simulink model "sampleModel2403_pp_difftest"  (R2018a)
settings: Solver=VariableStepAuto  StartTime=0.0  StopTime=10.0  RelTol=1e-3
undefined symbols (not defined in the file): DiscIntNeverNeededParam, sigbuilder_block
libraries: simulink x128
(part 3 of 3)

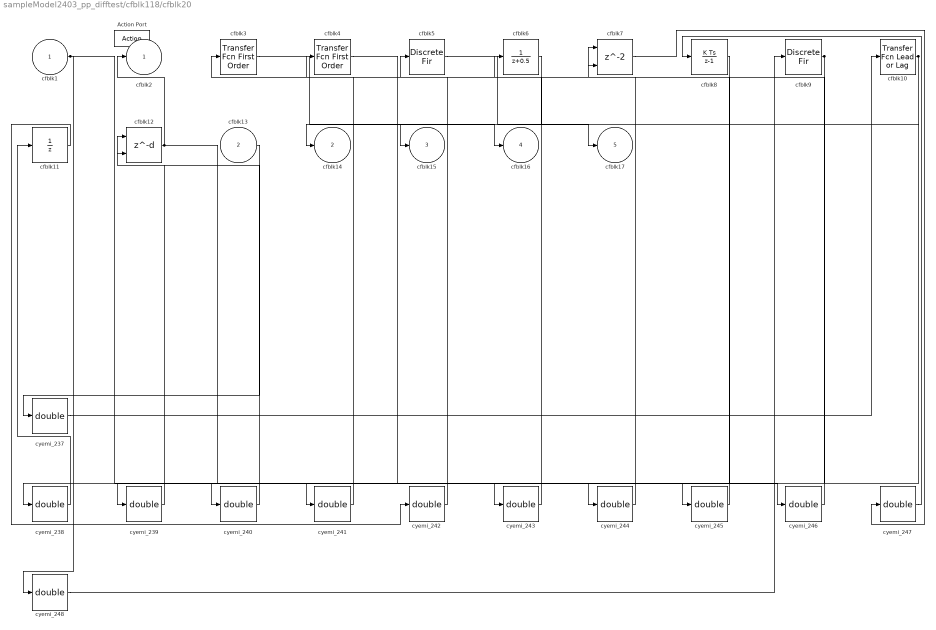
== system sampleModel2403_pp_difftest/cfblk118/cfblk20 ==
  cfblk1 : Inport
  cfblk13 : Inport  Port=2
  Action Port : ActionPort  ActionType=else
  cfblk10 : simulink/Discrete/Transfer Fcn Lead or Lag  PoleZ=0.95  ZeroZ=0.75  ICPrevOutput=0.0  ICPrevInput=0.0  DoSatur=off
      settings: SourceProductName=Simulink  SourceProductBaseCode=SL
  cfblk11 : UnitDelay  SampleTime=-1
  cfblk12 : Delay  DelayLengthSource=Input port
      settings: InputPortMap=u0,p1
  cfblk3 : simulink/Discrete/Transfer Fcn First Order  PoleZ=0.95  ICPrevOutput=0.0  DoSatur=off
      settings: SourceProductName=Simulink
  cfblk4 : simulink/Discrete/Transfer Fcn First Order  PoleZ=0.95  ICPrevOutput=0.0  DoSatur=off
      settings: SourceProductName=Simulink
  cfblk5 : DiscreteFir
  cfblk6 : DiscreteTransferFcn
  cfblk7 : Delay  ShowEnablePort=on
      settings: InputPortMap=u0,e6
  cfblk8 : DiscreteIntegrator  SampleTime=-1  OutDataTypeStr=double  ICPrevOutput=DiscIntNeverNeededParam  ICPrevScaledInput=DiscIntNeverNeededParam
  cfblk9 : DiscreteFir
  cyemi_{237..248} (12 alike) : DataTypeConversion  OutDataTypeStr=double
  cfblk2 : Outport
  cfblk14 : Outport  Port=2
  cfblk15 : Outport  Port=3
  cfblk16 : Outport  Port=4
  cfblk17 : Outport  Port=5
  wires:
  cfblk12/1 -> cfblk2/1, cyemi_243/1
  cfblk5/1 -> cfblk17/1
  cfblk3/1 -> cfblk16/1
  cfblk9/1 -> cyemi_239/1, cyemi_240/1, cyemi_241/1
  cfblk6/1 -> cfblk14/1
  cfblk10/1 -> cfblk15/1, cyemi_245/1
  cfblk1/1 -> cyemi_238/1, cyemi_246/1
  cyemi_237/1 -> cfblk10/1
  cfblk13/1 -> cyemi_237/1
  cyemi_238/1 -> cfblk11/1
  cyemi_239/1 -> cfblk12/1
  cyemi_240/1 -> cfblk12/2
  cyemi_241/1 -> cfblk3/1
  cyemi_242/1 -> cfblk4/1
  cfblk11/1 -> cyemi_242/1
  cyemi_243/1 -> cfblk5/1
  cyemi_244/1 -> cfblk6/1
  cfblk4/1 -> cyemi_244/1
  cyemi_245/1 -> cfblk7/1
  cyemi_246/1 -> cfblk7/2
  cyemi_247/1 -> cfblk8/1
  cfblk7/1 -> cyemi_247/1
  cyemi_248/1 -> cfblk9/1
  cfblk8/1 -> cyemi_248/1

== system sampleModel2403_pp_difftest/cfblk123/cfblk17 ==
  cfblk1 : Inport
  Action Port : ActionPort  ActionType=then
  cfblk10 : Delay
  cfblk3 : simulink/Discrete/Transfer Fcn Lead or Lag  PoleZ=0.95  ZeroZ=0.75  ICPrevOutput=0.0  ICPrevInput=0.0  DoSatur=off
      settings: SourceProductName=Simulink  SourceProductBaseCode=SL
  cfblk4 : UnitDelay  SampleTime=-1
  cfblk5 : simulink/Discrete/Transfer Fcn First Order  PoleZ=0.95  ICPrevOutput=0.0  DoSatur=off
      settings: SourceProductName=Simulink
  cfblk6 : simulink/Discrete/Transfer Fcn First Order  PoleZ=0.95  ICPrevOutput=0.0  DoSatur=off
      settings: SourceProductName=Simulink
  cfblk7 : DiscreteStateSpace  SampleTime=-1
  cfblk8 : simulink/Continuous/PID Controller  Controller=PID  TimeDomain=Discrete-time  SampleTime=-1  IntegratorMethod=Forward Euler  FilterMethod=Forward Euler  Form=Parallel  UseFilter=on  ControllerParametersSource=internal  P=1  I=1  D=0  N=100  InitialConditionSource=internal  InitialConditionForIntegrator=0  InitialConditionForFilter=0  ExternalReset=none  LimitOutput=off  UpperSaturationLimit=inf  LowerSaturationLimit=-inf  LinearizeAsGain=off  AntiWindupMode=none  Kb=1  TrackingMode=off  Kt=1  PParamMin=[]  PParamMax=[]  IParamMin=[]  IParamMax=[]  DParamMin=[]  DParamMax=[]  NParamMin=[]  NParamMax=[]  KbParamMin=[]  KbParamMax=[]  KtParamMin=[]  KtParamMax=[]  POutMin=[]  POutMax=[]  IOutMin=[]  IOutMax=[]  DOutMin=[]  DOutMax=[]  NOutMin=[]  NOutMax=[]  KbOutMin=[]  KbOutMax=[]  KtOutMin=[]  KtOutMax=[]  IntegratorOutMin=[]  IntegratorOutMax=[]  FilterOutMin=[]  FilterOutMax=[]  SumOutMin=[]  SumOutMax=[]  SumI1OutMin=[]  SumI1OutMax=[]  SumI2OutMin=[]  SumI2OutMax=[]  SumI3OutMin=[]  SumI3OutMax=[]  SumDOutMin=[]  SumDOutMax=[]  SaturationOutMin=[]  SaturationOutMax=[]  IntegratorContinuousStateAttributes=''  IntegratorStateMustResolveToSignalObject=off  IntegratorRTWStateStorageClass=Auto  FilterContinuousStateAttributes=''  FilterStateMustResolveToSignalObject=off  FilterRTWStateStorageClass=Auto  DifferentiatorICPrevScaledInput=0  DifferentiatorOutMin=[]  DifferentiatorOutMax=[]  FilterDiffOutCoefMin=[]  FilterDiffOutCoefMax=[]  SumDenOutMin=[]  SumDenOutMax=[]  SumNumOutMin=[]  SumNumOutMax=[]  ReciprocalOutMin=[]  ReciprocalOutMax=[]  DivideOutMin=[]  DivideOutMax=[]  TunerSelectOption=Transfer Function Based (PID Tuner App)
  cyemi_{334..340} (7 alike) : DataTypeConversion  OutDataTypeStr=double
  cfblk2 : Outport
  cfblk9 : Outport  Port=2
  wires:
  cfblk4/1 -> cfblk2/1
  cfblk6/1 -> cyemi_335/1, cyemi_339/1
  cfblk8/1 -> cfblk9/1
  cyemi_334/1 -> cfblk10/1
  cfblk7/1 -> cyemi_334/1
  cyemi_335/1 -> cfblk3/1
  cyemi_336/1 -> cfblk4/1
  cfblk1/1 -> cyemi_336/1
  cyemi_337/1 -> cfblk5/1
  cfblk3/1 -> cyemi_337/1
  cyemi_338/1 -> cfblk6/1
  cfblk10/1 -> cyemi_338/1
  cyemi_339/1 -> cfblk7/1
  cyemi_340/1 -> cfblk8/1
  cfblk5/1 -> cyemi_340/1

== system sampleModel2403_pp_difftest/cfblk123/cfblk18 ==
  cfblk1 : Inport
  cfblk9 : Inport  Port=2
  cfblk10 : Inport  Port=3
  cfblk11 : Inport  Port=4
  Action Port : ActionPort  ActionType=else
  cfblk14 : Delay
  cfblk3 : DiscreteStateSpace  SampleTime=-1
  cfblk4 : DiscreteFir
  cfblk5 : simulink/Discrete/Difference  ICPrevInput=0.0  OutMin=[]  OutMax=[]  OutDataTypeStr=double  OutputDataTypeScalingMode=double  OutDataType=fixdt(1, 16)  OutScaling=2^-10  DoSatur=off
  cfblk6 : DiscreteStateSpace  SampleTime=-1
  cfblk7 : Delay  ShowEnablePort=on
      settings: InputPortMap=u0,e6
  cfblk8 : simulink/Discrete/Difference  ICPrevInput=0.0  OutMin=[]  OutMax=[]  OutDataTypeStr=double  OutputDataTypeScalingMode=double  OutDataType=fixdt(1, 16)  OutScaling=2^-10  DoSatur=off
  cyemi_{345..352} (8 alike) : DataTypeConversion  OutDataTypeStr=double
  cfblk2 : Outport
  cfblk12 : Outport  Port=2
  cfblk13 : Outport  Port=3
  wires:
  cfblk5/1 -> cfblk13/1
  cfblk11/1 -> cfblk2/1
  cfblk6/1 -> cfblk12/1, cyemi_352/1
  cyemi_345/1 -> cfblk14/1
  cfblk7/1 -> cyemi_345/1
  cyemi_346/1 -> cfblk3/1
  cfblk1/1 -> cyemi_346/1
  cyemi_347/1 -> cfblk4/1
  cfblk14/1 -> cyemi_347/1
  cyemi_348/1 -> cfblk5/1
  cfblk9/1 -> cyemi_348/1
  cyemi_349/1 -> cfblk6/1
  cfblk3/1 -> cyemi_349/1
  cyemi_350/1 -> cfblk7/1
  cfblk4/1 -> cyemi_350/1
  cyemi_351/1 -> cfblk7/2
  cfblk10/1 -> cyemi_351/1
  cyemi_352/1 -> cfblk8/1

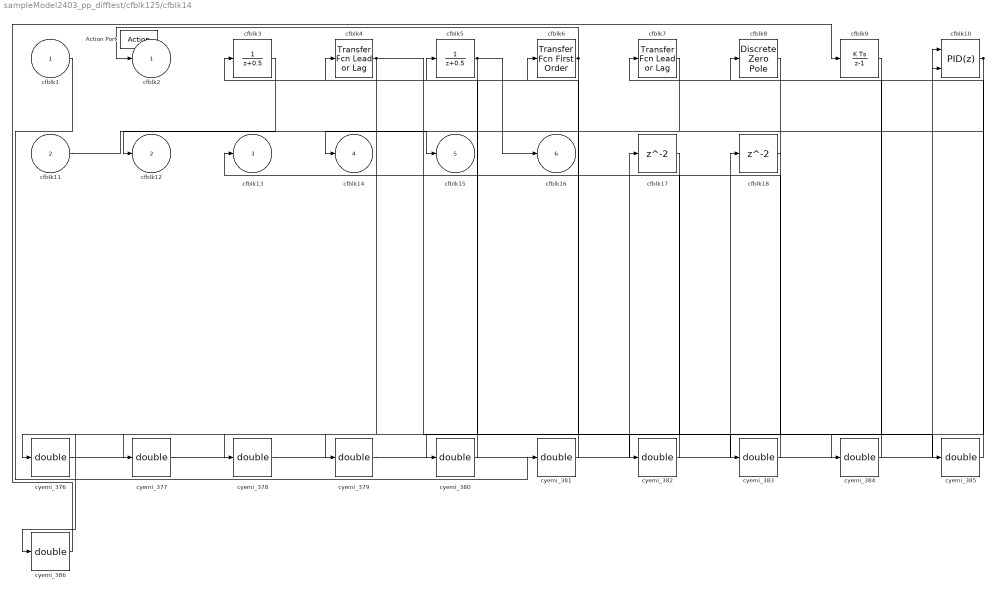
== system sampleModel2403_pp_difftest/cfblk125/cfblk14 ==
  cfblk1 : Inport
  cfblk11 : Inport  Port=2
  Action Port : ActionPort  ActionType=then
  cfblk10 : simulink/Continuous/PID Controller (2DOF)  Controller=PID  TimeDomain=Discrete-time  SampleTime=-1  IntegratorMethod=Forward Euler  FilterMethod=Forward Euler  Form=Parallel  UseFilter=on  ControllerParametersSource=internal  P=1  I=1  D=0  N=100  b=1  c=1  InitialConditionSource=internal  InitialConditionForIntegrator=0  InitialConditionForFilter=0  ExternalReset=none  LimitOutput=off  UpperSaturationLimit=inf  LowerSaturationLimit=-inf  LinearizeAsGain=off  AntiWindupMode=none  Kb=1  TrackingMode=off  Kt=1  PParamMin=[]  PParamMax=[]  IParamMin=[]  IParamMax=[]  DParamMin=[]  DParamMax=[]  NParamMin=[]  NParamMax=[]  bParamMin=[]  bParamMax=[]  cParamMin=[]  cParamMax=[]  KbParamMin=[]  KbParamMax=[]  KtParamMin=[]  KtParamMax=[]  POutMin=[]  POutMax=[]  IOutMin=[]  IOutMax=[]  DOutMin=[]  DOutMax=[]  NOutMin=[]  NOutMax=[]  bOutMin=[]  bOutMax=[]  cOutMin=[]  cOutMax=[]  KbOutMin=[]  KbOutMax=[]  KtOutMin=[]  KtOutMax=[]  IntegratorOutMin=[]  IntegratorOutMax=[]  FilterOutMin=[]  FilterOutMax=[]  SumOutMin=[]  SumOutMax=[]  Sum1OutMin=[]  Sum1OutMax=[]  Sum2OutMin=[]  Sum2OutMax=[]  Sum3OutMin=[]  Sum3OutMax=[]  SumI1OutMin=[]  SumI1OutMax=[]  SumI2OutMin=[]  SumI2OutMax=[]  SumI3OutMin=[]  SumI3OutMax=[]  SumDOutMin=[]  SumDOutMax=[]  SaturationOutMin=[]  SaturationOutMax=[]  IntegratorContinuousStateAttributes=''  IntegratorStateMustResolveToSignalObject=off  IntegratorRTWStateStorageClass=Auto  FilterContinuousStateAttributes=''  FilterStateMustResolveToSignalObject=off  FilterRTWStateStorageClass=Auto  DifferentiatorICPrevScaledInput=0  DifferentiatorOutMin=[]  DifferentiatorOutMax=[]  FilterDiffOutCoefMin=[]  FilterDiffOutCoefMax=[]  SumDenOutMin=[]  SumDenOutMax=[]  SumNumOutMin=[]  SumNumOutMax=[]  ReciprocalOutMin=[]  ReciprocalOutMax=[]  DivideOutMin=[]  DivideOutMax=[]  TunerSelectOption=Transfer Function Based (PID Tuner App)
  cfblk17 : Delay
  cfblk18 : Delay
  cfblk3 : DiscreteTransferFcn
  cfblk4 : simulink/Discrete/Transfer Fcn Lead or Lag  PoleZ=0.95  ZeroZ=0.75  ICPrevOutput=0.0  ICPrevInput=0.0  DoSatur=off
      settings: SourceProductName=Simulink  SourceProductBaseCode=SL
  cfblk5 : DiscreteTransferFcn
  cfblk6 : simulink/Discrete/Transfer Fcn First Order  PoleZ=0.95  ICPrevOutput=0.0  DoSatur=off
      settings: SourceProductName=Simulink
  cfblk7 : simulink/Discrete/Transfer Fcn Lead or Lag  PoleZ=0.95  ZeroZ=0.75  ICPrevOutput=0.0  ICPrevInput=0.0  DoSatur=off
      settings: SourceProductName=Simulink  SourceProductBaseCode=SL
  cfblk8 : DiscreteZeroPole  Poles=[0 0.5]  Gain=1  SampleTime=-1
  cfblk9 : DiscreteIntegrator  SampleTime=-1  OutDataTypeStr=double  ICPrevOutput=DiscIntNeverNeededParam  ICPrevScaledInput=DiscIntNeverNeededParam
  cyemi_{376..386} (11 alike) : DataTypeConversion  OutDataTypeStr=double
  cfblk2 : Outport
  cfblk12 : Outport  Port=2
  cfblk13 : Outport  Port=3
  cfblk14 : Outport  Port=4
  cfblk15 : Outport  Port=5
  cfblk16 : Outport  Port=6
  wires:
  cfblk3/1 -> cfblk12/1
  cfblk8/1 -> cfblk13/1
  cfblk11/1 -> cfblk15/1
  cfblk6/1 -> cfblk2/1, cyemi_378/1
  cfblk10/1 -> cfblk14/1, cyemi_379/1, cyemi_383/1
  cfblk5/1 -> cfblk16/1, cyemi_376/1
  cfblk4/1 -> cyemi_385/1, cyemi_386/1
  cyemi_376/1 -> cfblk10/1
  cyemi_377/1 -> cfblk10/2
  cfblk17/1 -> cyemi_377/1
  cyemi_378/1 -> cfblk17/1
  cyemi_379/1 -> cfblk18/1
  cyemi_380/1 -> cfblk3/1
  cfblk7/1 -> cyemi_380/1
  cyemi_381/1 -> cfblk4/1
  cfblk1/1 -> cyemi_381/1
  cyemi_382/1 -> cfblk5/1
  cfblk18/1 -> cyemi_382/1
  cyemi_383/1 -> cfblk6/1
  cyemi_384/1 -> cfblk7/1
  cfblk9/1 -> cyemi_384/1
  cyemi_385/1 -> cfblk8/1
  cyemi_386/1 -> cfblk9/1

== system sampleModel2403_pp_difftest/cfblk125/cfblk15 ==
  cfblk1 : Inport
  Action Port : ActionPort  ActionType=else
  cfblk10 : Delay
  cfblk3 : simulink/Continuous/PID Controller  Controller=PID  TimeDomain=Discrete-time  SampleTime=-1  IntegratorMethod=Forward Euler  FilterMethod=Forward Euler  Form=Parallel  UseFilter=on  ControllerParametersSource=internal  P=1  I=1  D=0  N=100  InitialConditionSource=internal  InitialConditionForIntegrator=0  InitialConditionForFilter=0  ExternalReset=none  LimitOutput=off  UpperSaturationLimit=inf  LowerSaturationLimit=-inf  LinearizeAsGain=off  AntiWindupMode=none  Kb=1  TrackingMode=off  Kt=1  PParamMin=[]  PParamMax=[]  IParamMin=[]  IParamMax=[]  DParamMin=[]  DParamMax=[]  NParamMin=[]  NParamMax=[]  KbParamMin=[]  KbParamMax=[]  KtParamMin=[]  KtParamMax=[]  POutMin=[]  POutMax=[]  IOutMin=[]  IOutMax=[]  DOutMin=[]  DOutMax=[]  NOutMin=[]  NOutMax=[]  KbOutMin=[]  KbOutMax=[]  KtOutMin=[]  KtOutMax=[]  IntegratorOutMin=[]  IntegratorOutMax=[]  FilterOutMin=[]  FilterOutMax=[]  SumOutMin=[]  SumOutMax=[]  SumI1OutMin=[]  SumI1OutMax=[]  SumI2OutMin=[]  SumI2OutMax=[]  SumI3OutMin=[]  SumI3OutMax=[]  SumDOutMin=[]  SumDOutMax=[]  SaturationOutMin=[]  SaturationOutMax=[]  IntegratorContinuousStateAttributes=''  IntegratorStateMustResolveToSignalObject=off  IntegratorRTWStateStorageClass=Auto  FilterContinuousStateAttributes=''  FilterStateMustResolveToSignalObject=off  FilterRTWStateStorageClass=Auto  DifferentiatorICPrevScaledInput=0  DifferentiatorOutMin=[]  DifferentiatorOutMax=[]  FilterDiffOutCoefMin=[]  FilterDiffOutCoefMax=[]  SumDenOutMin=[]  SumDenOutMax=[]  SumNumOutMin=[]  SumNumOutMax=[]  ReciprocalOutMin=[]  ReciprocalOutMax=[]  DivideOutMin=[]  DivideOutMax=[]  TunerSelectOption=Transfer Function Based (PID Tuner App)
  cfblk4 : Delay  ShowEnablePort=on
      settings: InputPortMap=u0,e6
  cfblk5 : DiscreteZeroPole  Poles=[0 0.5]  Gain=1  SampleTime=-1
  cfblk6 : DiscreteStateSpace  SampleTime=-1
  cfblk7 : simulink/Discrete/Transfer Fcn Lead or Lag  PoleZ=0.95  ZeroZ=0.75  ICPrevOutput=0.0  ICPrevInput=0.0  DoSatur=off
      settings: SourceProductName=Simulink  SourceProductBaseCode=SL
  cyemi_{388..394} (7 alike) : DataTypeConversion  OutDataTypeStr=double
  cfblk2 : Outport
  cfblk8 : Outport  Port=2
  cfblk9 : Outport  Port=3
  wires:
  cfblk7/1 -> cfblk2/1, cyemi_388/1
  cfblk3/1 -> cfblk9/1, cyemi_392/1
  cfblk4/1 -> cfblk8/1
  cfblk6/1 -> cyemi_391/1, cyemi_394/1
  cyemi_388/1 -> cfblk10/1
  cyemi_389/1 -> cfblk3/1
  cfblk10/1 -> cyemi_389/1
  cyemi_390/1 -> cfblk4/1
  cfblk1/1 -> cyemi_390/1
  cyemi_391/1 -> cfblk4/2
  cyemi_392/1 -> cfblk5/1
  cyemi_393/1 -> cfblk6/1
  cfblk5/1 -> cyemi_393/1
  cyemi_394/1 -> cfblk7/1
